simulink model "cdif"  (R2018a)
settings: Solver=VariableStepAuto  StartTime=0.0  StopTime=10.0  RelTol=1e-3
values from neighbouring files (symbols this model uses):
  A = [ -2 1;  1 1 ]    [sol.m]
  B = [ 1; 2 ]    [sol.m]
  C = [ 2 1 ]    [sol.m]
libraries: fuzblock x1
settings Model: Creator=daniel  LastModifiedBy=daniel

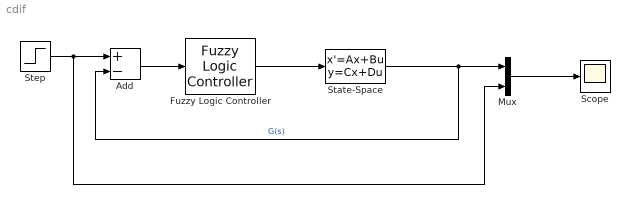
== system cdif ==
  Add : Sum  Inputs=+-
  Fuzzy Logic Controller : fuzblock/Fuzzy Logic  Controller  FIS='tipper.fis'  OutputSampleNumber=101  DataType=double  FuzzifiedInputs=off  RuleFiringStrengths=off  RuleOutputs=off  AggregatedOutputs=off  SimulateUsing=Interpreted execution  OutOfRangeInputValueMessage=warning  NoRuleFiredMessage=warning  EmptyOutputFuzzySetMessage=warning
  Mux : Mux  Inputs=2
  Scope : Scope
  State-Space : StateSpace  A=A  B=B  C=C  D=0  InitialCondition=0
  Step : Step  SampleTime=0
  wires:
  Mux/1 -> Scope/1
  Fuzzy Logic Controller/1 -> State-Space/1
  State-Space/1 -> Add/2, Mux/1  "G(s)"
  Step/1 -> Mux/2, Add/1
  Add/1 -> Fuzzy Logic Controller/1
